simulink model "lqr_control"  (R2019b)
settings: Solver=FixedStepAuto  StartTime=0.0  StopTime=inf  FixedStep=0.01  RelTol=1e-3
values from neighbouring files (symbols this model uses):
  K = K / 1.8    [control_parameter.m]
  K_c = K_c / 3    [control_parameter.m]
  sys_c_d = c2d(sys_c,Ts)    [control_parameter.m]
libraries: robotlib x8, simulink x2, dsparch4 x1
settings Model: Creator=shunya  LastModifiedBy=shunya
settings OptimizationCC: EnhancedBackFolding=on  PassReuseOutputArgsAs=Individual arguments  ZeroExternalMemoryAtStartup=off  ZeroInternalMemoryAtStartup=off  MaxStackSize=64  OptimizeBlockOrder=speed  DifferentSizesBufferReuse=on  OptimizationCustomize=off  EfficientTunableParamExpr=on
settings DebuggingCC: ParameterTunabilityLossMsg=error
settings HardwareCC: ProdBitPerPointer=32  ProdBitPerSizeT=32  ProdBitPerPtrDiffT=32  ProdLargestAtomicFloat=None  ProdIntDivRoundTo=Undefined  ProdEndianess=Unspecified  ProdWordSize=32  ProdHWDeviceType=Generic->Unspecified (assume 32-bit Generic)
settings SFSimCC: MATLABDynamicMemAlloc=off
settings RTWCC: SystemTargetFile=ert.tlc  HardwareBoard=Robot Operating System (ROS)  TLCOptions="-aInlineSetEventsForThisBaseRateFcn=TLC_FALSE -aSuppressMultiTaskScheduler=TLC_FALSE  -aRateBasedStepFcn=0"  TemplateMakefile=ert_default_tmf  GenerateReport=on  Toolchain=Catkin  IncludeHyperlinkInReport=on  LaunchReport=on  TargetLang=C++  GenerateTraceInfo=on  GenerateTraceReport=on  GenerateTraceReportSl=on  GenerateTraceReportSf=on  GenerateTraceReportEml=on
settings CodeAppCC: ForceParamTrailComments=on  IgnoreCustomStorageClasses=off  OperatorAnnotations=on  SimulinkDataObjDesc=on  SFDataObjDesc=on  InsertBlockDesc=on

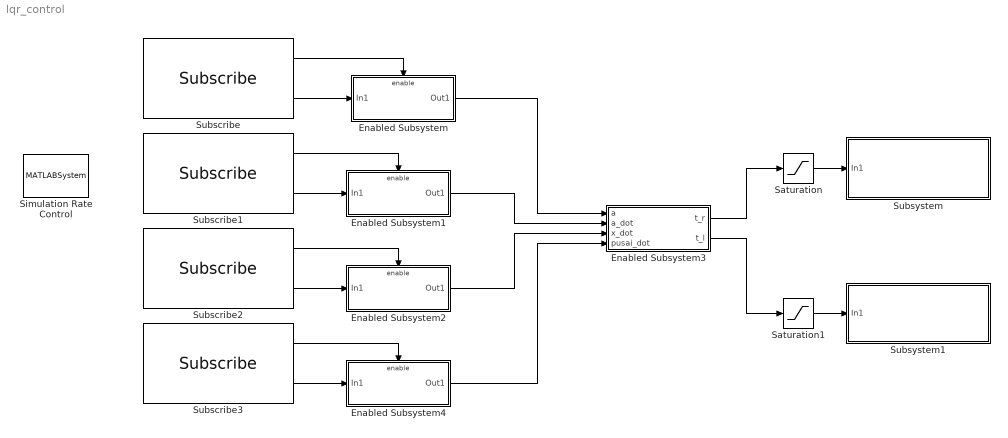
== system lqr_control ==
  Enabled Subsystem : Subsystem  TreatAsAtomicUnit=on
  Enabled Subsystem1 : Subsystem  TreatAsAtomicUnit=on
  Enabled Subsystem2 : Subsystem  TreatAsAtomicUnit=on
  Enabled Subsystem3 : Subsystem  TreatAsAtomicUnit=on
  Enabled Subsystem4 : Subsystem  TreatAsAtomicUnit=on
  Saturation : Saturate  UpperLimit=2  LowerLimit=-2
  Saturation1 : Saturate  UpperLimit=2  LowerLimit=-2
  Simulation Rate Control : MATLABSystem  System=ExampleHelperSimulationRateControl  SampleTime=0.01
      mask Type: ExampleHelperSimulationRateControl
      mask Display: disp('Rate Control');
  Subscribe : robotlib/Subscribe  topicSource=Specify your own  topic=/balance_state_angle  messageType=std_msgs/Float64  sampleTime=0.01  messageQueueLength=1
      settings: SourceProductName=ROS Toolbox
  Subscribe1 : robotlib/Subscribe  topicSource=Select from ROS network  topic=/balance_state_angular  messageType=std_msgs/Float64  sampleTime=0.01  messageQueueLength=1
      settings: SourceProductName=ROS Toolbox
  Subscribe2 : robotlib/Subscribe  topicSource=Select from ROS network  topic=/balance_state_velocity  messageType=std_msgs/Float64  sampleTime=0.01  messageQueueLength=1
      settings: SourceProductName=ROS Toolbox
  Subscribe3 : robotlib/Subscribe  topicSource=Select from ROS network  topic=/balance_state_pusai  messageType=std_msgs/Float64  sampleTime=0.01  messageQueueLength=1
      settings: SourceProductName=ROS Toolbox
  Subsystem : Subsystem
  Subsystem1 : Subsystem
  wires:
  Subscribe/2 -> Enabled Subsystem/1(In1)
  Subscribe/1 -> Enabled Subsystem/Enable
  Subscribe1/1 -> Enabled Subsystem1/Enable
  Subscribe1/2 -> Enabled Subsystem1/1(In1)
  Subscribe2/2 -> Enabled Subsystem2/1(In1)
  Subscribe2/1 -> Enabled Subsystem2/Enable
  Subscribe3/1 -> Enabled Subsystem4/Enable
  Subscribe3/2 -> Enabled Subsystem4/1(In1)
  Enabled Subsystem/1(Out1) -> Enabled Subsystem3/1(a)
  Enabled Subsystem1/1(Out1) -> Enabled Subsystem3/2(a_dot)
  Enabled Subsystem2/1(Out1) -> Enabled Subsystem3/3(x_dot)
  Enabled Subsystem4/1(Out1) -> Enabled Subsystem3/4(pusai_dot)
  Saturation/1 -> Subsystem/1(In1)
  Enabled Subsystem3/1(t_r) -> Saturation/1
  Saturation1/1 -> Subsystem1/1(In1)
  Enabled Subsystem3/2(t_l) -> Saturation1/1

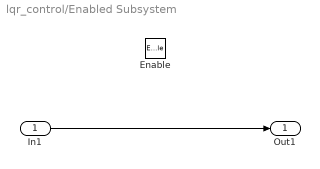
== system lqr_control/Enabled Subsystem ==
  In1 : Inport
  Enable : EnablePort
  Out1 : Outport
  wires:
  In1/1 -> Out1/1

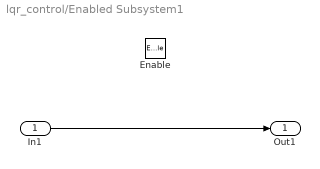
== system lqr_control/Enabled Subsystem1 ==
  In1 : Inport
  Enable : EnablePort
  Out1 : Outport
  wires:
  In1/1 -> Out1/1

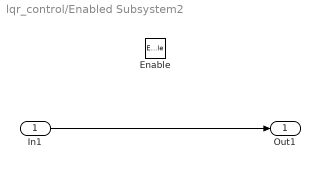
== system lqr_control/Enabled Subsystem2 ==
  In1 : Inport
  Enable : EnablePort
  Out1 : Outport
  wires:
  In1/1 -> Out1/1

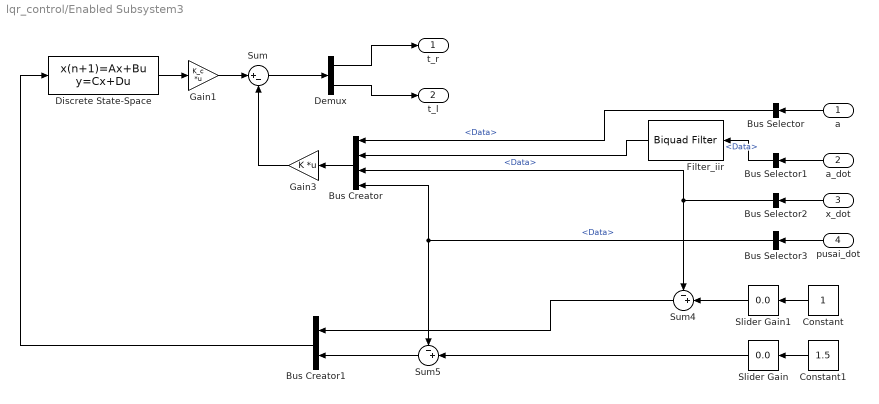
== system lqr_control/Enabled Subsystem3 ==
  a : Inport
  a_dot : Inport  Port=2
  x_dot : Inport  Port=3
  pusai_dot : Inport  Port=4
  Bus Creator : BusCreator  Inputs=4
  Bus Creator1 : BusCreator  Inputs=2
  Bus Selector{,1..3} (4 alike) : BusSelector  OutputSignals=Data
  Constant : Constant
  Constant1 : Constant  Value=1.5
  Demux : Demux  Outputs=2
  Discrete State-Space : DiscreteStateSpace  A=sys_c_d.A  B=sys_c_d.B  C=sys_c_d.C  D=sys_c_d.D  SampleTime=-1
  Filter_iir : dsparch4/Biquad Filter  Tag=BlockMethodSubSystem  FilterSource=Dialog parameters  CoeffSource=Specify via dialog  FilterObject=BQF  IIRFiltStruct=Direct form II  BiQuadCoeffs=[1 -1.39091039225363255 1 1 -1.74775050195611481 0.786332153473716988;1 -1.83447076363198858 1 1 -1.85416271752759898 0.950035013452580901]  ScaleValues=[0.542276961837810934;0.0602971640489207844;1]  IC=0  ICnum=0  ICden=0  a0Flag=Warning  optimizeScaleValues=on  ScaleValueMode=Specify via input port (g)  InputProcessing=Columns as channels (frame based)  roundingMode=Floor  overflowMode=off  scaleValueFracLength=14  denProdOutputFracLength=30  denAccumFracLength=30  secondMemoryFracLength=15
      settings: SourceProductName=DSP System Toolbox
  Gain1 : Gain  Gain=K_c  Multiplication=Matrix(K*u) (u vector)
  Gain3 : Gain  Gain=K  Multiplication=Matrix(K*u) (u vector)
  Slider Gain : simulink/Math Operations/Slider Gain  gain=0.0  low=-1  high=1
  Slider Gain1 : simulink/Math Operations/Slider Gain  gain=0.0  low=-1  high=1
  Sum : Sum  Inputs=|+-
  Sum4 : Sum  Inputs=-+|
  Sum5 : Sum  Inputs=-+|
  t_r : Outport
  t_l : Outport  Port=2
  wires:
  a/1 -> Bus Selector/1
  pusai_dot/1 -> Bus Selector3/1
  x_dot/1 -> Bus Selector2/1
  a_dot/1 -> Bus Selector1/1
  Bus Selector/1 -> Bus Creator/1  "<Data>"
  Bus Selector3/1 -> Bus Creator/4, Sum5/1  "<Data>"
  Bus Selector2/1 -> Bus Creator/3, Sum4/1  "<Data>"
  Bus Creator/1 -> Gain3/1
  Constant/1 -> Slider Gain1/1
  Constant1/1 -> Slider Gain/1
  Demux/1 -> t_r/1
  Demux/2 -> t_l/1
  Sum4/1 -> Bus Creator1/1
  Sum5/1 -> Bus Creator1/2
  Bus Creator1/1 -> Discrete State-Space/1
  Discrete State-Space/1 -> Gain1/1
  Gain3/1 -> Sum/2
  Sum/1 -> Demux/1
  Slider Gain/1 -> Sum5/2
  Slider Gain1/1 -> Sum4/2
  Gain1/1 -> Sum/1
  Bus Selector1/1 -> Filter_iir/1  "<Data>"
  Filter_iir/1 -> Bus Creator/2

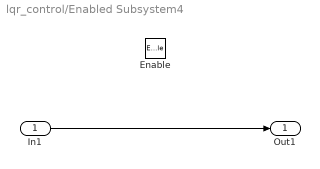
== system lqr_control/Enabled Subsystem4 ==
  In1 : Inport
  Enable : EnablePort
  Out1 : Outport
  wires:
  In1/1 -> Out1/1

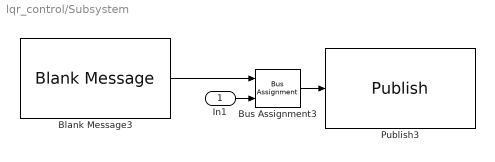
== system lqr_control/Subsystem ==
  In1 : Inport
  Blank Message3 : robotlib/Blank Message  messageClass=Message  entityType=std_msgs/Float64  messageType=std_msgs/Float64  SampleTime=-1
      settings: SourceProductName=ROS Toolbox
  Bus Assignment3 : BusAssignment  AssignedSignals=Data
  Publish3 : robotlib/Publish  topicSource=Select from ROS network  topic=/wheel_leg/right_wheel_effort_controller/command  messageType=std_msgs/Float64  messageQueueLength=5
      settings: SourceProductName=ROS Toolbox
  wires:
  Blank Message3/1 -> Bus Assignment3/1
  Bus Assignment3/1 -> Publish3/1
  In1/1 -> Bus Assignment3/2

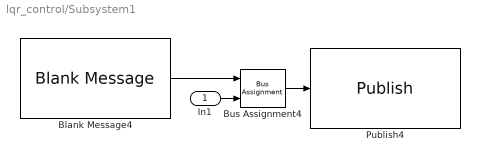
== system lqr_control/Subsystem1 ==
  In1 : Inport
  Blank Message4 : robotlib/Blank Message  messageClass=Message  entityType=std_msgs/Float64  messageType=std_msgs/Float64  SampleTime=-1
      settings: SourceProductName=ROS Toolbox
  Bus Assignment4 : BusAssignment  AssignedSignals=Data
  Publish4 : robotlib/Publish  topicSource=Select from ROS network  topic=/wheel_leg/left_wheel_effort_controller/command  messageType=std_msgs/Float64  messageQueueLength=5
      settings: SourceProductName=ROS Toolbox
  wires:
  Bus Assignment4/1 -> Publish4/1
  In1/1 -> Bus Assignment4/2
  Blank Message4/1 -> Bus Assignment4/1
